simulink model "controller"  (R2022b)
settings: Solver=FixedStepAuto  StartTime=0.0  StopTime=10.0  FixedStep=1/100  RelTol=1e-3
undefined symbols (not defined in the file): MAX_SPEED_BACKWARD, MAX_SPEED_FORWARD, MAX_TORQUE, MAX_TORQUE_REVERSE
settings Model: Creator=DAUIN-Win10  LastModifiedBy=jacoposini
settings DebuggingCC: UnconnectedInputMsg=warning  UnconnectedOutputMsg=warning  UnconnectedLineMsg=warning
settings ModelReferenceCC: EnableRefExpFcnMdlSchedulingChecks=on
settings RTWCC: DLArmComputeVersion=19.05

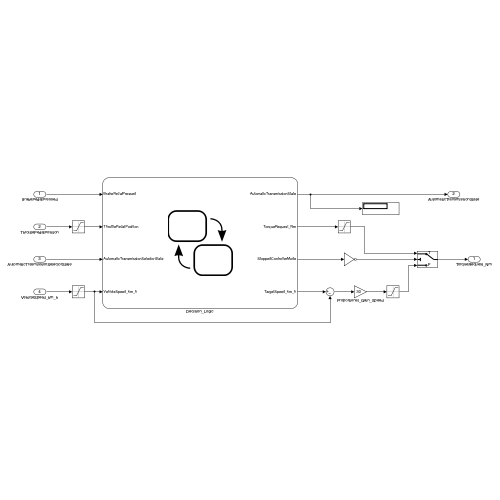
[thumbnail: Simulink's stored preview of the top-level diagram]
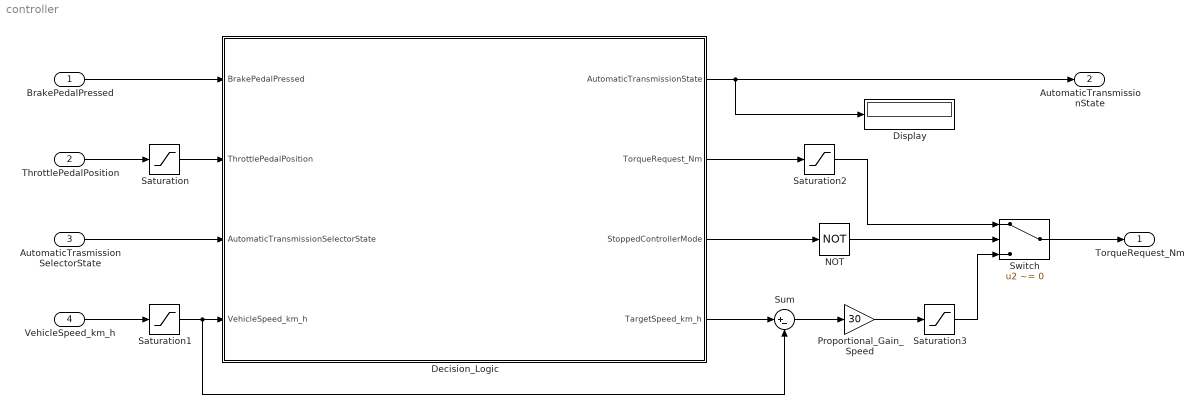
== system controller ==
  BrakePedalPressed : Inport  OutDataTypeStr=boolean
  ThrottlePedalPosition : Inport  Port=2  OutDataTypeStr=single
  AutomaticTrasmissionSelectorState : Inport  Port=3  OutDataTypeStr=Enum: TransmissionState
  VehicleSpeed_km_h : Inport  Port=4  OutDataTypeStr=single  Unit=km/h
  Decision_Logic : Stateflow chart  TreatAsAtomicUnit=on
  Display : Display
  NOT : Logic  Operator=NOT  IconShape=distinctive  AllPortsSameDT=off  OutDataTypeStr=boolean
  Proportional_Gain_Speed : Gain  Gain=30
  Saturation : Saturate  UpperLimit=1  LowerLimit=0
  Saturation1 : Saturate  UpperLimit=MAX_SPEED_FORWARD  LowerLimit=-MAX_SPEED_BACKWARD
  Saturation2 : Saturate  UpperLimit=MAX_TORQUE  LowerLimit=-MAX_TORQUE
  Saturation3 : Saturate  UpperLimit=MAX_TORQUE  LowerLimit=-MAX_TORQUE
  Sum : Sum  Inputs=|+-
  Switch : Switch  Criteria=u2 ~= 0  OutDataTypeStr=single  SaturateOnIntegerOverflow=off  InputSameDT=off
  TorqueRequest_Nm : Outport  OutDataTypeStr=single  Unit=N*m
  AutomaticTransmissionState : Outport  Port=2  OutDataTypeStr=Enum: TransmissionState
  wires:
  BrakePedalPressed/1 -> Decision_Logic/1(BrakePedalPressed)
  ThrottlePedalPosition/1 -> Saturation/1
  AutomaticTrasmissionSelectorState/1 -> Decision_Logic/3(AutomaticTransmissionSelectorState)
  VehicleSpeed_km_h/1 -> Saturation1/1
  Decision_Logic/2(TorqueRequest_Nm) -> Saturation2/1
  Decision_Logic/1(AutomaticTransmissionState) -> Display/1, AutomaticTransmissionState/1
  Saturation/1 -> Decision_Logic/2(ThrottlePedalPosition)
  Saturation1/1 -> Sum/2, Decision_Logic/4(VehicleSpeed_km_h)
  Decision_Logic/3(StoppedControllerMode) -> NOT/1
  Saturation2/1 -> Switch/1
  Switch/1 -> TorqueRequest_Nm/1
  Decision_Logic/4(TargetSpeed_km_h) -> Sum/1
  Sum/1 -> Proportional_Gain_Speed/1
  Saturation3/1 -> Switch/3
  Proportional_Gain_Speed/1 -> Saturation3/1
  NOT/1 -> Switch/2

== stateflow chart controller/Decision_Logic ==
  state Init
    en:
    AutomaticTransmissionState = Park;
    TorqueRequest_Nm = 0.0;
  state Reverse
    en:
    AutomaticTransmissionState = Reverse;
    TorqueRequest_Nm = 0.0;
    du:
    TorqueRequest_Nm = ThrottlePedalPosition * -MAX_TORQUE_REVERSE;
  state StoppedReverse
    en:
    StoppedControllerMode = true;
    state Stop
      en:
      TargetSpeed_km_h  = -0.0;
    state Start
      en:
      TargetSpeed_km_h  = -5;
    (default) -> StoppedReverse.Stop
    StoppedReverse.Start -> StoppedReverse.Stop : [BrakePedalPressed == true]
    StoppedReverse.Stop -> (junction 75) : [BrakePedalPressed == true]
    (junction 75) -> StoppedReverse.Start : [BrakePedalPressed == false]
  state Neutral
    en:
    AutomaticTransmissionState = Neutral;
    TorqueRequest_Nm = 0.0;
  state ParkReleaseState
    en:
    AutomaticTransmissionState = Park;
    ParkRelease = true;
    TorqueRequest_Nm = 0.0;
  state Stopped
    en:
    StoppedControllerMode = true;
    state Stop
      en:
      TargetSpeed_km_h  = 0.0;
    state Start
      en:
      TargetSpeed_km_h  = 5;
    (default) -> Stopped.Stop
    Stopped.Start -> Stopped.Stop : [BrakePedalPressed == true]
    Stopped.Stop -> (junction 63) : [BrakePedalPressed == true]
    (junction 63) -> Stopped.Start : [BrakePedalPressed == false]
  state Drive
    en:
    AutomaticTransmissionState = Drive;
    StoppedControllerMode = false;
  state Brake
    en:
    AutomaticTransmissionState = Brake;
    StoppedControllerMode = false;
    du:
    TorqueRequest_Nm = 0.0;
  (default) -> Init
  Reverse -> StoppedReverse [order 3] : [VehicleSpeed_km_h > - 3.0 &&...
      | BrakePedalPressed == true && ...
      | ThrottlePedalPosition < (1.0/10.0)]
  Init -> Reverse [order 2] : [AutomaticTransmissionSelectorState == Reverse && ...
      |  BrakePedalPressed == true]
  StoppedReverse -> Reverse : [VehicleSpeed_km_h > -3.5 && ...
      | TargetSpeed_km_h < -2.0 || ...
      | ThrottlePedalPosition > (1.0/10.0)]
  Reverse -> Init [order 1] : [AutomaticTransmissionSelectorState == Park && ...
      |  BrakePedalPressed == true && ...
      | abs(VehicleSpeed_km_h) < 0.5 ]
  Init -> ParkReleaseState [order 1] : [AutomaticTransmissionSelectorState == Park && ...
      | ParkRelease == true]
  Init -> Brake [order 5] : [AutomaticTransmissionSelectorState == Brake && ...
      |  BrakePedalPressed == true && ...
      | VehicleSpeed_km_h > -0.5 ]
  ParkReleaseState -> Init
  Init -> Drive [order 4] : [AutomaticTransmissionSelectorState == Drive && ...
      |  BrakePedalPressed == true && ...
      | VehicleSpeed_km_h > -0.5 ]
  Init -> Neutral [order 3] : [AutomaticTransmissionSelectorState == Neutral && ...
      |  BrakePedalPressed == true]
  Reverse -> Neutral [order 2] : [AutomaticTransmissionSelectorState == Neutral]
  Neutral -> Reverse [order 1] : [AutomaticTransmissionSelectorState == Reverse && ...
      |  (BrakePedalPressed == true || ...
      | VehicleSpeed_km_h < 5.0) ]
  Brake -> Neutral [order 2] : [AutomaticTransmissionSelectorState == Neutral || ...
      | AutomaticTransmissionSelectorState == Reverse]
  Neutral -> Drive [order 2] : [AutomaticTransmissionSelectorState == Drive && ...
      |  (BrakePedalPressed == true || ...
      | VehicleSpeed_km_h > -5) ]
  Drive -> Neutral [order 1] : [AutomaticTransmissionSelectorState == Neutral || ...
      | AutomaticTransmissionSelectorState == Reverse]
  Drive -> Drive [order 3] : [BrakePedalPressed == false]...
      | {TorqueRequest_Nm = ThrottlePedalPosition * MAX_TORQUE;}
  Stopped -> Drive [order 1] : [(VehicleSpeed_km_h > 3.5 && ...
      | TargetSpeed_km_h > 2.0) || ...
      | ThrottlePedalPosition > (1.0/10.0)]
  Drive -> Drive [order 4] : [BrakePedalPressed == true]...
      | {TorqueRequest_Nm = 0.0;}
  Drive -> Stopped [order 5] : [VehicleSpeed_km_h < 3.0 &&...
      | BrakePedalPressed == true]
  Drive -> Brake [order 2] : [AutomaticTransmissionSelectorState == Brake && ...
      | (ThrottlePedalPosition > (1.0/3.0) || BrakePedalPressed == true)]
  Brake -> Drive [order 1] : [AutomaticTransmissionSelectorState == Drive && ...
      | (ThrottlePedalPosition < (1.0/3.0) || BrakePedalPressed == true)]
  Brake -> Stopped [order 6] : [ThrottlePedalPosition < 0.05 && ...
      | VehicleSpeed_km_h < 3.0]
  Stopped -> Brake [order 2] : [ThrottlePedalPosition > (1.0/3.0)]
  Brake -> Brake [order 4] : [BrakePedalPressed == false && ThrottlePedalPosition > (1.0/3.0)]...
      | {TorqueRequest_Nm = MAX_TORQUE * (3.0/2.0) * (ThrottlePedalPosition - 1.0/3.0);}
  Brake -> Brake [order 3] : [ThrottlePedalPosition < (1.0/3.0) && VehicleSpeed_km_h > 0.0]...
      | {TorqueRequest_Nm = -MAX_TORQUE * (1.0- 3.0*ThrottlePedalPosition);}
  Brake -> Brake [order 5] : [BrakePedalPressed == true && ThrottlePedalPosition > (1.0/3.0)]...
      | {TorqueRequest_Nm = 0.0;}
  data: BrakePedalPressed input boolean; ThrottlePedalPosition input single; AutomaticTransmissionSelectorState input Enum: TransmissionState; VehicleSpeed_km_h input single; AutomaticTransmissionState output Enum: TransmissionState size=1; TorqueRequest_Nm output single; ParkRelease local boolean =false; MAX_TORQUE parameter; MAX_TORQUE_REVERSE parameter; StoppedControllerMode output boolean; TargetSpeed_km_h output single
